simulink model "Vehicle_coordinate_transfer"  (R2021a)
settings: configuration reference "AION_IDS_Speedgoat" (kept outside this file)
libraries: simulink x1
Description:
  | 地球平面坐标点转换到车辆坐标系
settings Model: DataDictionary=Vehicle_Coordinate_Transfer.sldd  Creator=xinrui  LastModifiedBy=Administrator
settings ConfigSetRef: SourceName=AION_IDS_Speedgoat

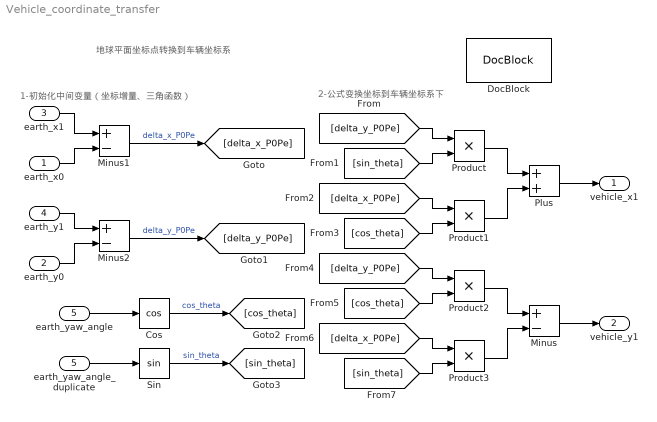
== system Vehicle_coordinate_transfer ==
  note: 2-公式变换坐标到车辆坐标系下
  note: 地球平面坐标点转换到车辆坐标系
  note: 1-初始化中间变量（坐标增量、三角函数）
  earth_x0 : Inport  Description=车辆当前点P0在地球平面坐标系下的x坐标，实数，m。  OutDataTypeStr=double  PortDimensions=1
  earth_y0 : Inport  Description=车辆当前点P0在地球平面坐标系下的x坐标，实数，m。  Port=2  OutDataTypeStr=double  PortDimensions=1
  earth_x1 : Inport  Description=指定点Pe在地球平面坐标系下的x坐标，实数，m。  Port=3  OutDataTypeStr=double  PortDimensions=1
  earth_y1 : Inport  Description=指定点Pe在地球平面坐标系下的y坐标，实数，m。  Port=4  OutDataTypeStr=double  PortDimensions=1
  earth_yaw_angle : Inport  Description=车辆在地球平面坐标系下的横摆角，实数，rad。  Port=5  OutDataTypeStr=double  PortDimensions=1
  Cos : Trigonometry  Description=计算车辆当前横摆角的余弦值。  Operator=cos
  DocBlock : simulink/Model-Wide Utilities/DocBlock  DocumentType=HTML  mask(DocBlock){}
      mask Display:
      | plot([.8 0 0 1 1 .8 .8 1],[1 1 0 0 .8 1 .8 .8]);
      | text(.5,.6,'CHANGELOG','horizontalalignment','center');
      | text(.95,.05,get_param(gcb,'DocumentType'),'verticalalignment','bottom','horizontalalignment','right');
  Minus : Sum  Description=按照公式将地球平面坐标系下的Pe点变换到车辆坐标系下的Pv点。  Inputs=+-
  Minus1 : Sum  Description=计算指定点Pe与车辆当前点P0之间的x坐标增量。  Inputs=+-
  Minus2 : Sum  Description=计算指定点Pe与车辆当前点P0之间的y坐标增量。  Inputs=+-
  Plus : Sum  Description=按照公式将地球平面坐标系下的Pe点变换到车辆坐标系下的Pv点。
  Product{,1..3} (4 alike) : Product
  Sin : Trigonometry  Description=计算车辆当前横摆角的正弦值。
  earth_yaw_angle_duplicate : InportShadow  Port=5  OutDataTypeStr=double  PortDimensions=1
  vehicle_x1 : Outport  Description=指定点Pe变换到车辆坐标系下的Pv点x坐标，实数，m。
  vehicle_y1 : Outport  Description=指定点Pe变换到车辆坐标系下的Pv点y坐标，实数，m。  Port=2
  wires:
  earth_x1/1 -> Minus1/1
  earth_y1/1 -> Minus2/1
  earth_x0/1 -> Minus1/2
  Minus1/1 -> [delta_x_P0Pe]  "delta_x_P0Pe"
  earth_y0/1 -> Minus2/2
  Minus2/1 -> [delta_y_P0Pe]  "delta_y_P0Pe"
  Cos/1 -> [cos_theta]  "cos_theta"
  earth_yaw_angle/1 -> Cos/1
  Sin/1 -> [sin_theta]  "sin_theta"
  earth_yaw_angle_duplicate/1 -> Sin/1
  [delta_y_P0Pe] -> Product/1
  [sin_theta] -> Product/2
  [delta_x_P0Pe] -> Product1/1
  [cos_theta] -> Product1/2
  Product/1 -> Plus/1
  Product1/1 -> Plus/2
  Plus/1 -> vehicle_x1/1
  [sin_theta] -> Product3/2
  [delta_x_P0Pe] -> Product3/1
  [cos_theta] -> Product2/2
  [delta_y_P0Pe] -> Product2/1
  Product2/1 -> Minus/1
  Product3/1 -> Minus/2
  Minus/1 -> vehicle_y1/1
